simulink model "untitled3"  (R2023b)
settings: Solver=VariableStepAuto  StartTime=0.0  StopTime=10.0  RelTol=1e-3
undefined symbols (not defined in the file or in its folder): r_k, Td, Tf, Ti

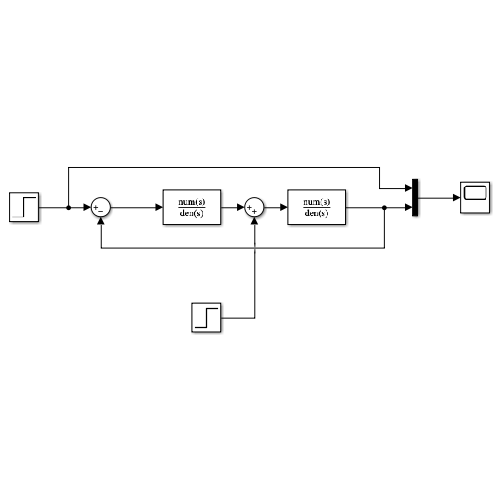
[thumbnail: Simulink's stored preview of the top-level diagram]
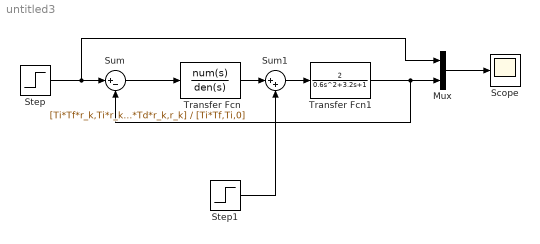
== system untitled3 ==
  Mux : Mux  Inputs=2
  Scope : Scope
  Step : Step  SampleTime=0
  Step1 : Step  SampleTime=0
  Sum : Sum  Inputs=|+-
  Sum1 : Sum  Inputs=|++
  Transfer Fcn : TransferFcn  Numerator=[Ti*Tf*r_k,Ti*r_k+Tf*r_k+Ti*Td*r_k,r_k]  Denominator=[Ti*Tf,Ti,0]
  Transfer Fcn1 : TransferFcn  Numerator=[2]  Denominator=[0.6 3.2 1]
  wires:
  Step/1 -> Mux/1, Sum/1
  Sum/1 -> Transfer Fcn/1
  Transfer Fcn1/1 -> Sum/2, Mux/2
  Mux/1 -> Scope/1
  Transfer Fcn/1 -> Sum1/1
  Sum1/1 -> Transfer Fcn1/1
  Step1/1 -> Sum1/2
